simulink model "MehanickiSistem2012B"  (R2012b)
settings: Solver=ode45  SolverMode=SingleTasking  StartTime=0.0  StopTime=10  RelTol=1e-3
undefined symbols (not defined in the file): k, m, z
libraries: fuzblock x1, simulink x1
settings Model: CovMetricSettings=dwe  CovHtmlReporting=off  covSaveCumulativeToWorkspaceVar=off  CovSaveSingleToWorkspaceVar=off  CovExternalEMLEnable=on  Creator=Aldin  LastModifiedBy=Aldin
settings DataIOCC: LimitDataPoints=off  SaveFormat=StructureWithTime  ReturnWorkspaceOutputs=on
settings OptimizationCC: ExpressionDepthLimit=128
settings DebuggingCC: UnderspecifiedInitializationDetection=Simplified  MergeDetectMultiDrivingBlocksExec=error  SolverPrmCheckMsg=none  FrameProcessingCompatibilityMsg=error  StateNameClashWarn=none  SFUnexpectedBacktrackingDiag=error  SFNoUnconditionalDefaultTransitionDiag=error
settings HardwareCC: ProdBitPerPointer=64  ProdLargestAtomicFloat=Float  ProdIntDivRoundTo=Zero  ProdEndianess=LittleEndian  ProdHWDeviceType=Specified
settings ModelReferenceCC: PropagateSignalLabelsOutOfModel=on
settings SFSimCC: SimUseLocalCustomCode=on
settings RTWCC: RTWUseLocalCustomCode=on
settings CodeAppCC: CustomSymbolStrType=$N$R$M_T
settings GRTTargetCC: CodeReplacementLibrary=C99 (ISO)

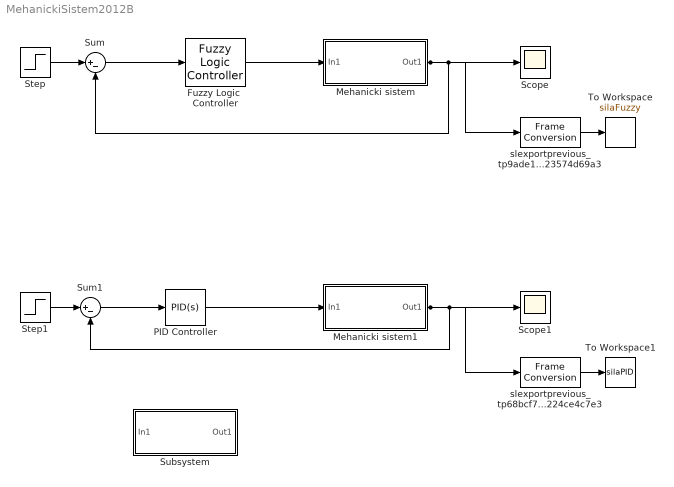
== system MehanickiSistem2012B ==
  Fuzzy Logic  Controller : fuzblock/Fuzzy Logic  Controller  FIS=Mehs
  Mehanicki sistem : Subsystem
  Mehanicki sistem1 : Subsystem
  PID Controller : simulink/Continuous/PID Controller  Controller=PID  Form=Parallel  TimeDomain=Continuous-time  SampleTime=-1  IntegratorMethod=Forward Euler  FilterMethod=Forward Euler  ControllerParametersSource=internal  P=7.80036144704785  I=0.829836993663022  D=13.2061899071902  UseFilter=on  N=166.910508167407  InitialConditionSource=internal  InitialConditionForIntegrator=0  InitialConditionForFilter=0  DifferentiatorICPrevScaledInput=0  ExternalReset=none  TrackingMode=off  Kt=1  LimitOutput=off  UpperSaturationLimit=inf  LowerSaturationLimit=-inf  LinearizeAsGain=on  AntiWindupMode=none  Kb=1  POutMin=[]  POutMax=[]  IOutMin=[]  IOutMax=[]  DOutMin=[]  DOutMax=[]  NOutMin=[]  NOutMax=[]  SumOutMin=[]  SumOutMax=[]  SaturationOutMin=[]  SaturationOutMax=[]  PParamMin=[]  PParamMax=[]  IParamMin=[]  IParamMax=[]  DParamMin=[]  DParamMax=[]  NParamMin=[]  NParamMax=[]  KbParamMin=[]  KbParamMax=[]  KtParamMin=[]  KtParamMax=[]  KbOutMin=[]  KbOutMax=[]  KtOutMin=[]  KtOutMax=[]  IntegratorOutMin=[]  IntegratorOutMax=[]  FilterOutMin=[]  FilterOutMax=[]  SumI1OutMin=[]  SumI1OutMax=[]  SumI2OutMin=[]  SumI2OutMax=[]  SumI3OutMin=[]  SumI3OutMax=[]  SumDOutMin=[]  SumDOutMax=[]  DifferentiatorOutMin=[]  DifferentiatorOutMax=[]  IntegratorContinuousStateAttributes=''  IntegratorStateMustResolveToSignalObject=off  IntegratorRTWStateStorageClass=Auto  FilterContinuousStateAttributes=''  FilterStateMustResolveToSignalObject=off  FilterRTWStateStorageClass=Auto
  Scope : Scope
      settings: TimeRange=auto  LimitDataPoints=on  MaxDataPoints=5000  SaveToWorkspace=off  SaveName=ScopeData  YMin=-12.70519  YMax=114.34671  SampleTime=-1
  Scope1 : Scope
      settings: TimeRange=auto  LimitDataPoints=on  MaxDataPoints=5000  SaveToWorkspace=off  YMin=-14.10417  YMax=126.93751  SampleTime=-1
  Step : Step  Time=0  SampleTime=0
  Step1 : Step  Time=0  After=100  SampleTime=0
  Subsystem : Subsystem
  Sum : Sum  Inputs=|+-
  Sum1 : Sum  Inputs=|+-
  To Workspace : ToWorkspace  VariableName=silaFuzzy  SampleTime=-1
  To Workspace1 : ToWorkspace  VariableName=silaPID  SampleTime=-1
  slexportprevious_tp68bcf7c0_3ffd_434e_987b_a5224ce4c7e3 : FrameConversion  OutFrame=Sample-based
  slexportprevious_tp9ade1618_1513_47cc_9329_0523574d69a3 : FrameConversion  OutFrame=Sample-based
  wires:
  Mehanicki sistem/1(Out1) -> Sum/2, Scope/1, slexportprevious_tp9ade1618_1513_47cc_9329_0523574d69a3/1
  Sum/1 -> Fuzzy Logic  Controller/1
  Step/1 -> Sum/1
  Mehanicki sistem1/1(Out1) -> Sum1/2, Scope1/1, slexportprevious_tp68bcf7c0_3ffd_434e_987b_a5224ce4c7e3/1
  Step1/1 -> Sum1/1
  Fuzzy Logic  Controller/1 -> Mehanicki sistem/1(In1)
  PID Controller/1 -> Mehanicki sistem1/1(In1)
  Sum1/1 -> PID Controller/1
  slexportprevious_tp9ade1618_1513_47cc_9329_0523574d69a3/1 -> To Workspace/1
  slexportprevious_tp68bcf7c0_3ffd_434e_987b_a5224ce4c7e3/1 -> To Workspace1/1

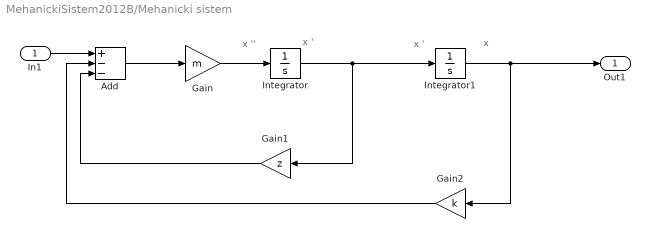
== system MehanickiSistem2012B/Mehanicki sistem ==
  note: x '
  note: x
  note: x '
  note: x ''
  In1 : Inport
  Add : Sum  Inputs=+--
  Gain : Gain  Gain=m
  Gain1 : Gain  Gain=z
  Gain2 : Gain  Gain=k
  Integrator : Integrator
  Integrator1 : Integrator
  Out1 : Outport
  wires:
  Integrator/1 -> Gain1/1, Integrator1/1
  Integrator1/1 -> Gain2/1, Out1/1
  In1/1 -> Add/1
  Add/1 -> Gain/1
  Gain/1 -> Integrator/1
  Gain1/1 -> Add/3
  Gain2/1 -> Add/2

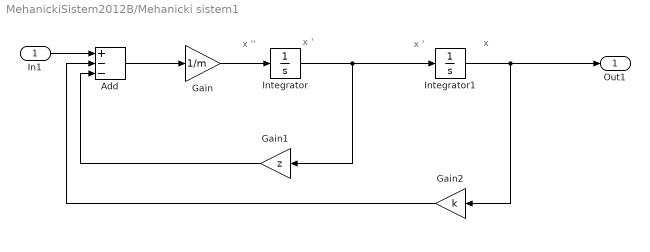
== system MehanickiSistem2012B/Mehanicki sistem1 ==
  note: x '
  note: x
  note: x '
  note: x ''
  In1 : Inport
  Add : Sum  Inputs=+--
  Gain : Gain  Gain=1/m
  Gain1 : Gain  Gain=z
  Gain2 : Gain  Gain=k
  Integrator : Integrator
  Integrator1 : Integrator
  Out1 : Outport
  wires:
  Integrator/1 -> Gain1/1, Integrator1/1
  Integrator1/1 -> Gain2/1, Out1/1
  In1/1 -> Add/1
  Add/1 -> Gain/1
  Gain/1 -> Integrator/1
  Gain1/1 -> Add/3
  Gain2/1 -> Add/2

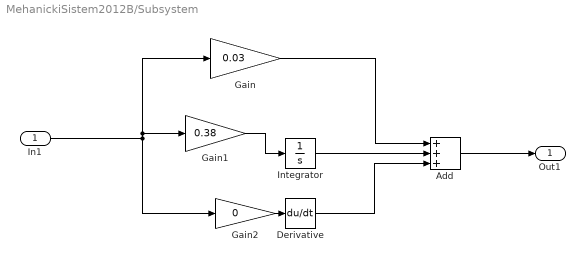
== system MehanickiSistem2012B/Subsystem ==
  In1 : Inport
  Add : Sum  Inputs=+++
  Derivative : Derivative
  Gain : Gain  Gain=0.03
  Gain1 : Gain  Gain=0.38
  Gain2 : Gain  Gain=0
  Integrator : Integrator
  Out1 : Outport
  wires:
  In1/1 -> Gain1/1, Gain/1, Gain2/1
  Gain/1 -> Add/1
  Integrator/1 -> Add/2
  Gain1/1 -> Integrator/1
  Gain2/1 -> Derivative/1
  Derivative/1 -> Add/3
  Add/1 -> Out1/1
